simulink model "Power_converter_new"  (R2018b)
settings: Solver=VariableStepAuto  StartTime=0.0  StopTime=6  RelTol=1e-3
model workspace (MAT data in the model file):
  Cripple1 = 0.1
  indripple = Simulink.Parameter
  indripple.Value = 0.001
  indripple.DataType = 'auto'
  indripple.DocUnits = 'H'
  indripple.Dimensions = [1 1]
undefined symbols (not defined in the file): sigbuilder_block
libraries: powerlib x29, simulink x2, powerlib_meascontrol x2
settings Model: OrderedModelArguments=off  Creator=Nicholas  LastModifiedBy=Joseph
settings SolverCC: ZeroCrossAlgorithm=Adaptive
settings DebuggingCC: IgnoredZcDiagnostic=none

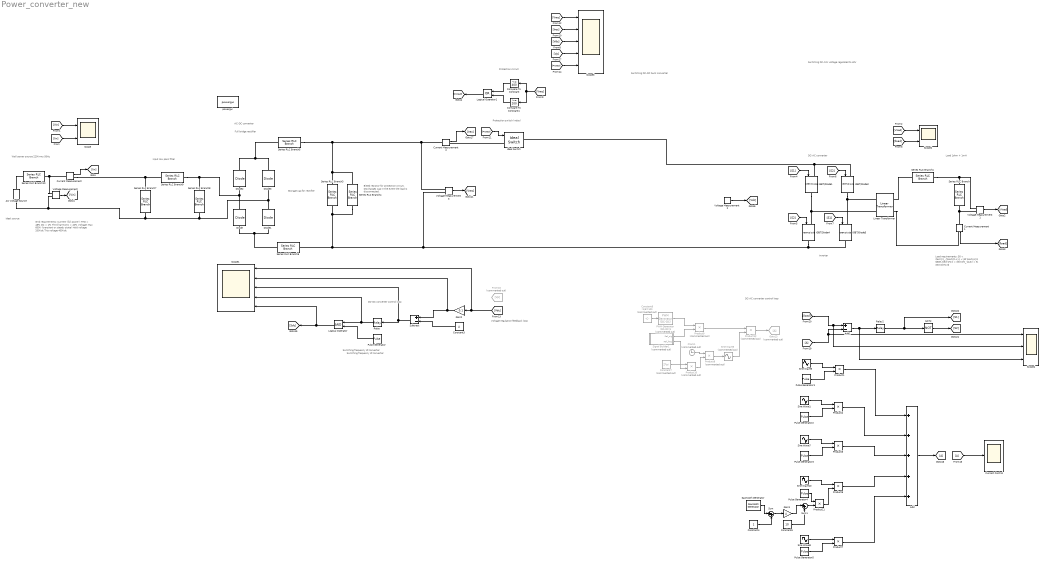
== system Power_converter_new ==
  note: Wall power source
      | 220Vrms 50Hz
  note: AC-DC converter
  note: Load
      | 1ohm + 1mH
  note: Load requirements:
      | $0 < \text{I}_{\text{R-L}} < 30 \text{A}$
      | $500\ \text{Hz} < \text{f}_{out} < 5\ \text{kHz}$
  note: Grid requirements:
      | Current (full power):
      | THD < 48%
      | DC < 1%
      | Third harmonic < 40%
      |
      | Voltage:
      | Max 600V (transient or steady state)
      | Hold voltage 200Vdc
      | Trip voltage 400Vdc
  note: DC-AC converter
  note: Full bridge rectifier
  note: Switching DC-DC buck converter
  note: Inverter
  note: Ideal source
  note: DC-DC converter control loop
  note: Voltage regulation feedback loop
  note: Switching frequency of converter
  note: DC-AC converter control loop
  note: Storage cap for rectifier
  note: Protection switch (relay)
  note: Protection circuit
  note: Bleed resistor for protection circuit.
      | Discharges cap in the event the load is disconnected.
  note: Switching DC-link voltage regulated to 40V
  note: Input low pass filter
  note: Switching frequency of converter
  AC Voltage Source : powerlib/Electrical Sources/AC Voltage Source  Amplitude=220*sqrt(2)  Phase=0  Frequency=50  SampleTime=0  Measurements=None  BusType=PQ  Pref=10e3  Qref=0  Qmin=-inf  Qmax=+inf
      settings: SourceProductName=Simscape Electrical
  Add : Sum  Inputs=5
  Add1 : Sum  Inputs=+-
  Clock1 : Clock  Commented=on
  Compare To Constant : simulink/Logic and Bit Operations/Compare To Constant  relop=<=  const=400  OutDataTypeStr=boolean
  Compare To Constant1 : simulink/Logic and Bit Operations/Compare To Constant  relop=>=  const=200  OutDataTypeStr=boolean
  Constant3 : Constant  Value=4
  Constant4 : Constant
  Constant5 : Constant  Value=10
  Constant6 : Constant  Commented=on  Value=(1/6)*100
  Constant7 : Constant  Commented=on  Value=2*pi
  "Current Control " : Scope
  Current Measurement : powerlib/Measurements/Current Measurement  PhasorSimulation=off  OutputType=Complex  PSBequivalent=0
      settings: SourceProductName=Simscape Electrical
  Current Measurement1 : powerlib/Measurements/Current Measurement  PhasorSimulation=off  OutputType=Complex  PSBequivalent=0
      settings: SourceProductName=Simscape Electrical
  Current Measurement2 : powerlib/Measurements/Current Measurement  PhasorSimulation=off  OutputType=Complex  PSBequivalent=0
      settings: SourceProductName=Simscape Electrical
  Diode{,1..3} (4 alike) : powerlib/Power Electronics/Diode  Ron=0.001  Lon=0  Vf=0.8  IC=0  UseSnubber=0  Rs=500  Cs=250e-9  Measurements=off
      settings: SourceProductName=Simscape Electrical
  From16 : From  Commented=on  GotoTag=Vp
  Gain1 : Gain  Gain=4
  Gain2 : Gain  Gain=0.1
  Goto13 : Goto  Commented=on
  IGBT/Diode{1..2,4..5} (4 alike) : powerlib/Power Electronics/IGBT//Diode  Ron=1e-3  Rs=1e5  Cs=inf  Measurements=off
      settings: SourceProductName=Simscape Electrical
  Ideal Switch : powerlib/Power Electronics/Ideal Switch  Ron=0.0001  Lon=0  IC=0  Rs=1e6  Cs=inf  Measurements=off
      settings: SourceProductName=Simscape Electrical
  Linear Transformer : powerlib/Elements/Linear Transformer  UNITS=SI  NominalPower=[ 250e6 50 ]  winding1=[7.35e+05 0 0]  winding2=[7.35e+05 0 0]  ThreeWindings=off  winding3=[3.15e+05 0.7938 0.084225]  RmLm=[Inf Inf]  Measurements=None  DataType=on
  Logical Operator : Logic  AllPortsSameDT=off  OutDataTypeStr=boolean
  Logical Operator1 : Logic  Operator=OR  AllPortsSameDT=off  OutDataTypeStr=boolean
  NOT2 : Logic  Operator=NOT  IconShape=distinctive  AllPortsSameDT=off  OutDataTypeStr=boolean
  PWM Generator (DC-DC)1 : powerlib_meascontrol/Pulse & Signal Generators/PWM Generator (DC-DC)  Commented=on  Fsw=5000  Ts=0
      settings: SourceProductName=Simscape Electrical
  Product{1..2,5..7,11} (6 alike) : Product
  Product{8..10,12} (4 alike) : Product  Commented=on
  Pulse Generator : DiscretePulseGenerator  PulseType=Time based  Period=1/40000  PulseWidth=50
  Pulse Generator1 : DiscretePulseGenerator  PulseType=Time based  Amplitude=3  Period=6  PulseWidth=1/6*100
  Pulse Generator2 : DiscretePulseGenerator  PulseType=Time based  Amplitude=20  Period=6  PulseWidth=1/3*100  PhaseDelay=1
  Pulse Generator3 : DiscretePulseGenerator  PulseType=Time based  Amplitude=10  Period=6  PulseWidth=1/3*100  PhaseDelay=3
  Pulse Generator4 : DiscretePulseGenerator  PulseType=Time based  Period=6  PulseWidth=1/12*100  PhaseDelay=5
  Pulse Generator5 : DiscretePulseGenerator  PulseType=Time based  Amplitude=18  Period=6  PulseWidth=1/12*100  PhaseDelay=5.5
  Relay : Relay  OnSwitchValue=0.0001  OffSwitchValue=-0.0001  OnOutputValue=0  OffOutputValue=1
  Relay2 : Relay  OnSwitchValue=0.5  OffSwitchValue=-0.5
  Sawtooth Generator : powerlib_meascontrol/Pulse & Signal Generators/Sawtooth Generator  Freq=1/0.5  Phase=0  Ts=0
      settings: SourceProductName=Simscape Electrical
  Scope : Scope  NumInputPorts=2
  Scope1 : Scope  NumInputPorts=5
  Scope2 : Scope  NumInputPorts=2
  Scope3 : Scope  NumInputPorts=5
  Scope4 : Scope  NumInputPorts=3
  Series RLC Branch : powerlib/Elements/Series RLC Branch  LConnTagsString=__new0  RConnTagsString=__new0  BranchType=RL  Resistance=1  Inductance=0.1e-3  SetiL0=off  InitialCurrent=0  Capacitance=1e-6  Setx0=off  InitialVoltage=0  Measurements=None
      settings: SourceProductName=Simscape Electrical
  Series RLC Branch1 : powerlib/Elements/Series RLC Branch  LConnTagsString=__new0  RConnTagsString=__new0  BranchType=C  Resistance=1  Inductance=0.1e-3  SetiL0=off  InitialCurrent=0  Capacitance=200E-6  Setx0=off  InitialVoltage=0  Measurements=None
      settings: SourceProductName=Simscape Electrical
  Series RLC Branch10 : powerlib/Elements/Series RLC Branch  LConnTagsString=__new0  RConnTagsString=__new0  BranchType=R  Resistance=0.001  Inductance=160E-6  SetiL0=off  InitialCurrent=0  Capacitance=0.002  Setx0=off  InitialVoltage=0  Measurements=None
      settings: SourceProductName=Simscape Electrical
  Series RLC Branch3 : powerlib/Elements/Series RLC Branch  LConnTagsString=__new0  RConnTagsString=__new0  BranchType=C  Resistance=1  Inductance=0.1e-3  SetiL0=off  InitialCurrent=0  Capacitance=200E-6  Setx0=off  InitialVoltage=0  Measurements=None
      settings: SourceProductName=Simscape Electrical
  Series RLC Branch4 : powerlib/Elements/Series RLC Branch  LConnTagsString=__new0  RConnTagsString=__new0  BranchType=R  Resistance=2E9  Inductance=0.1e-3  SetiL0=off  InitialCurrent=0  Capacitance=0.001  Setx0=off  InitialVoltage=0  Measurements=None
      settings: SourceProductName=Simscape Electrical
  Series RLC Branch5 : powerlib/Elements/Series RLC Branch  LConnTagsString=__new0  RConnTagsString=__new0  BranchType=L  Resistance=1  Inductance=160E-6  SetiL0=off  InitialCurrent=0  Capacitance=0.002  Setx0=off  InitialVoltage=0  Measurements=None
      settings: SourceProductName=Simscape Electrical
  Series RLC Branch6 : powerlib/Elements/Series RLC Branch  LConnTagsString=__new0  RConnTagsString=__new0  BranchType=L  Resistance=1  Inductance=160E-6  SetiL0=off  InitialCurrent=0  Capacitance=0.002  Setx0=off  InitialVoltage=0  Measurements=None
      settings: SourceProductName=Simscape Electrical
  Series RLC Branch7 : powerlib/Elements/Series RLC Branch  LConnTagsString=__new0  RConnTagsString=__new0  BranchType=C  Resistance=10E9  Inductance=0.1e-3  SetiL0=off  InitialCurrent=0  Capacitance=32E-6  Setx0=off  InitialVoltage=0  Measurements=None
      settings: SourceProductName=Simscape Electrical
  Series RLC Branch8 : powerlib/Elements/Series RLC Branch  LConnTagsString=__new0  RConnTagsString=__new0  BranchType=C  Resistance=1  Inductance=0.1e-3  SetiL0=off  InitialCurrent=0  Capacitance=32E-6  Setx0=off  InitialVoltage=0  Measurements=None
      settings: SourceProductName=Simscape Electrical
  Series RLC Branch9 : powerlib/Elements/Series RLC Branch  LConnTagsString=__new0  RConnTagsString=__new0  BranchType=L  Resistance=1  Inductance=1E-3  SetiL0=off  InitialCurrent=0  Capacitance=0.002  Setx0=off  InitialVoltage=0  Measurements=None
      settings: SourceProductName=Simscape Electrical
  Signal Builder1 : Subsystem  Tag=STV Subsys  Commented=on  LoadFcn=sigbuilder_block('load');  StartFcn=sigbuilder_block('start');  StopFcn=sigbuilder_block('stop');  ClipboardFcn=sigbuilder_block('clipboard');  mask(Sigbuilder block){tuvar=[0:10]}
      mask help: Simulink:masks:SigbuilderBlock_MD
      mask init:
      | if ~strcmp(get_param(bdroot(gcbh),'SimulationStatus'),'stopped') tuvar = sigbuilder_block('maskInit'); end
      settings: CopyFcn=sigbuilder_block('copy');  DeleteFcn=sigbuilder_block('delete');  ModelCloseFcn=sigbuilder_block('modelClose');  PreSaveFcn=sigbuilder_block('preSave');  PauseFcn=sigbuilder_block('pause');  ContinueFcn=sigbuilder_block('continue');  NameChangeFcn=sigbuilder_block('namechange');  OpenFcn=sigbuilder_block('open',[883.5 314.25 550.5 278.25 ]);  CloseFcn=sigbuilder_block('close');
      mask Display: plot(0, 0, 100, 100,[2, 2, 32, 32, 2], [68, 8, 8, 68, 68],[32, 2], [38, 38], [32, 19, 2],[53, 60, 44], [32, 17, 17, 2],[16, 16, 31, 31]);txt = getActiveGroup(gcbh);text(2, 100, txt,'verticalAlignment', 'top');
  Sine Wave1 : Sin  Frequency=5000*2*pi  SampleTime=0
  Sine Wave10 : Sin  Frequency=1000*2*pi  SampleTime=0
  Sine Wave3 : Sin  Commented=on  TimeSource=Use external signal  Amplitude=[1]  Bias=[0]  Frequency=[1]  Phase=[0]  SampleTime=0
  Sine Wave5 : Sin  Frequency=500*2*pi  SampleTime=0
  Sine Wave7 : Sin  Frequency=1000*2*pi  SampleTime=0
  Sine Wave8 : Sin  Frequency=1000*2*pi  SampleTime=0
  Subtract : Sum  Inputs=+-
  Sum : Sum  Inputs=|++
  Sum1 : Sum  Inputs=|++
  Voltage Measurement{,1..3} (4 alike) : powerlib/Measurements/Voltage Measurement  PhasorSimulation=off  OutputType=Complex  PSBequivalent=0
      settings: SourceProductName=Simscape Electrical
  powergui : powerlib/powergui  Priority=1  SimulationMode=Discrete  SampleTime=1E-5  frequency=60  Iterations=50  frequencyindice=0  Pbase=100e6  ErrMax=1e-4  UnitsV=kV  UnitsW=MW  buscounter=0  FunctionMessages=off  echomessages=off  EnableUseOfTLC=off  CurrentSourceSwitches=off  DisableSnubberDevices=off  DisableRonSwitches=off  DisableVfSwitches=off  DisplayEquations=off  SolverType=Tustin/Backward Euler (TBE)  Interpol=off  ExternalGateDelay=off  methode=off  Ts=100  x0status=blocks  SPID=on  SwTol=0  HookPort=off  RestoreLinks=warning  ResistiveCurrentMeasurement=off  Frange=[0:2:500]  Ylog=off  Xlog=on  ShowGrid=off  save=off  variable=ZData  structure=ScopeData  ZoomFFT=on  StartTime=0.41  cycles=4  DisplayStyle=2  fundamental=50  FreqAxis=off  MaxFrequency=10000  frequencyindicesteady=1  RmsSteady=1  display=off
  wires:
  Voltage Measurement/1 -> [Vin]
  Current Measurement/1 -> [Iin]
  Voltage Measurement1/1 -> [Vload]
  [Iin] -> Scope/2
  [Vin] -> Scope/1
  Current Measurement1/1 -> [Iload]
  [S2] -> IGBT/Diode2/1
  [S2] -> IGBT/Diode4/1
  [S1] -> IGBT/Diode1/1
  [S1] -> IGBT/Diode5/1
  [Vload] -> Scope2/1
  [Iload] -> Scope2/2
  Voltage Measurement3/1 -> [Vrec]
  [Vrec] -> Scope3/1
  Constant3/1 -> Subtract/2
  Current Measurement2/1 -> [Irec]
  [Iload] -> Scope4/2, Add1/1
  Sine Wave5/1 -> Product1/1
  Sum1/1 -> Product11/2
  Constant5/1 -> Sum1/2
  Product1/1 -> Add/1
  Product11/1 -> Product6/2
  Gain1/1 -> Sum1/1
  Constant4/1 -> Sum/2
  [A] -> Scope4/1, Add1/2
  Sawtooth Generator/1 -> Sum/1
  Product5/1 -> Add/3
  Add/1 -> [A]
  Sine Wave1/1 -> Product2/1
  Product7/1 -> Add/5
  Pulse Generator2/1 -> Product2/2
  Sum/1 -> Gain1/1
  Product6/1 -> Add/4
  Sine Wave8/1 -> Product7/1
  Pulse Generator3/1 -> Product5/2
  Sine Wave10/1 -> Product6/1
  Pulse Generator4/1 -> Product11/1
  Pulse Generator1/1 -> Product1/2
  Sine Wave7/1 -> Product5/1
  Pulse Generator5/1 -> Product7/2
  NOT2/1 -> [S2]
  Add1/1 -> Relay2/1, Scope4/3
  [Vdc] -> Scope3/3
  [Irec] -> Scope3/2
  Constant6/1 -> PWM Generator (DC-DC)1/1
  PWM Generator (DC-DC)1/1 -> Product9/1
  Signal Builder1/1(Ref_sig) -> Product9/2
  Product10/1 -> Product8/2
  Constant7/1 -> Product10/1
  Clock1/1 -> Product8/1
  Product8/1 -> Sine Wave3/1
  Signal Builder1/2(Ref_freq) -> Product10/2
  Product9/1 -> Product12/1
  Sine Wave3/1 -> Product12/2
  Product12/1 -> Goto13/1
  [Vdc] -> Scope1/1, Gain2/1
  Gain2/1 -> Scope1/2, Subtract/1
  Relay/1 -> Scope1/4, Logical Operator/1
  [Protect] -> Scope3/5
  Pulse Generator/1 -> Logical Operator/2
  Subtract/1 -> Relay/1, Scope1/3
  Compare To Constant1/1 -> Logical Operator1/2
  [Protect] -> Ideal Switch/1
  Compare To Constant/1 -> Logical Operator1/1
  [Vrec] -> Compare To Constant/1, Compare To Constant1/1
  Logical Operator1/1 -> [Protect]
  [A] -> "Current Control "/1
  [Vp] -> Scope3/4
  Product2/1 -> Add/2
  Relay2/1 -> [S1], NOT2/1
  Voltage Measurement2/1 -> [Vdc]
  Logical Operator/1 -> Scope1/5, [Sdc]
  connections:
  Voltage Measurement/LConn1 -- Current Measurement/LConn1 -- Series RLC Branch10/RConn1
  Current Measurement1/LConn1 -- Voltage Measurement1/LConn2 -- Series RLC Branch/RConn1
  Diode/RConn1 -- Series RLC Branch8/LConn1 -- Series RLC Branch9/RConn1 -- Diode2/LConn1
  IGBT/Diode1/RConn1 -- Linear Transformer/LConn2 -- IGBT/Diode4/LConn1
  Diode2/RConn1 -- Series RLC Branch5/LConn1 -- Diode3/RConn1
  Ideal Switch/LConn1 -- Current Measurement2/RConn1
  Diode3/LConn1 -- Series RLC Branch7/RConn1 -- Voltage Measurement/LConn2 -- AC Voltage Source/LConn1 -- Series RLC Branch8/RConn1 -- Diode1/RConn1
  Series RLC Branch9/LConn1 -- Current Measurement/RConn1 -- Series RLC Branch7/LConn1
  Series RLC Branch10/LConn1 -- AC Voltage Source/RConn1
  IGBT/Diode2/RConn1 -- Linear Transformer/LConn1 -- IGBT/Diode5/LConn1
  Series RLC Branch6/LConn1 -- Diode/LConn1 -- Diode1/LConn1
  Series RLC Branch4/LConn1 -- Series RLC Branch5/RConn1 -- Voltage Measurement3/LConn1 -- Current Measurement2/LConn1 -- Series RLC Branch3/LConn1
  IGBT/Diode4/RConn1 -- Voltage Measurement3/LConn2 -- Series RLC Branch6/RConn1 -- Series RLC Branch4/RConn1 -- Series RLC Branch3/RConn1 -- IGBT/Diode5/RConn1
  IGBT/Diode2/LConn1 -- Ideal Switch/RConn1 -- IGBT/Diode1/LConn1
  Series RLC Branch1/RConn1 -- Linear Transformer/RConn1
  Linear Transformer/RConn2 -- Current Measurement1/RConn1
  Series RLC Branch/LConn1 -- Series RLC Branch1/LConn1 -- Voltage Measurement1/LConn1

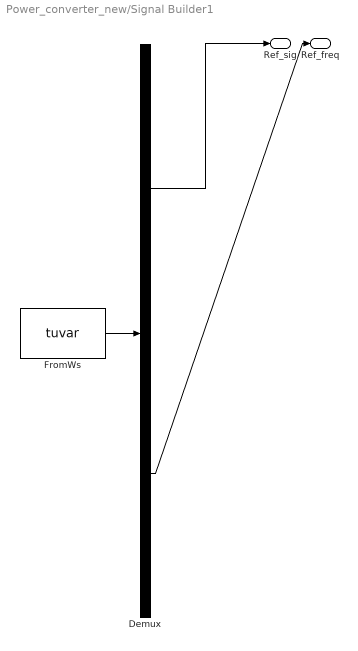
== system Power_converter_new/Signal Builder1 ==
  Demux : Demux  Tag=STV Demux  Outputs=2
  FromWs : FromWorkspace  Tag=STV FromWs  VariableName=tuvar  SampleTime=0
      SigBuilderData=|
      | common.afterFinalStr = 'Extrapolate'
      | common.sampleTime = 0
      | dataSet.timeRange = [0 10]
      | dataSet.name = 'Group 1'
      | sbobj.Groups.Name = 'Group 1'
      | sbobj.Groups.Signals(1).Name = 'Ref_sig'
      | sbobj.Groups.Signals(1).XData = [0 1 1 3 3 5 5.5 6 6 10]
      | sbobj.Groups.Signals(1).YData = [3 3 20 20 10 10 18 18 0 0]
      | sbobj.Groups.Signals(2).Name = 'Ref_freq'
      | sbobj.Groups.Signals(2).XData = [0 1 1 3 3 10]
      | sbobj.Groups.Signals(2).YData = [500 500 5000 5000 1000 1000]
  Ref_sig : Outport  Tag=STV Outport  VectorParamsAs1DForOutWhenUnconnected=on
  Ref_freq : Outport  Tag=STV Outport  Port=2  VectorParamsAs1DForOutWhenUnconnected=on
  wires:
  Demux/1 -> Ref_sig/1
  FromWs/1 -> Demux/1
  Demux/2 -> Ref_freq/1
